simulink subsystem "T_junction"  (R2022b)
settings: Solver=VariableStepAuto  StartTime=0.0  StopTime=10.0  RelTol=1e-3
values from neighbouring files (symbols this model uses):
  C0 = 1e-5    (= 1e-05)    [plantConstants.m]
  dt = 1/samplingRate    (= 0.025)    [plantConstants.m]    (also in sysID.m)
  L0 = L_aq    [plantConstants.m]
  ni = 3    [plantConstants.m]    (also in rls_.m = no; stateEstimator.m = size(Bp,2); toPhi_.m = no; wtMod_.m = no)
  no = 3    [plantConstants.m]    (also in rls_.m = size(phi,2); stateEstimator.m = size(Cp,1); sysID.m = length(outputs); theta2ss_.m = size(y0, 1))
  Rl0 = 0    [plantConstants.m]
  Rr0 = R_aq    [plantConstants.m]
  y_max = 500*ones(2*no, 1)    [plantConstants.m]
libraries: fl_lib x6, nesl_utility x4, simulink x1
settings Model: Creator=khqc  LastModifiedBy=khqc

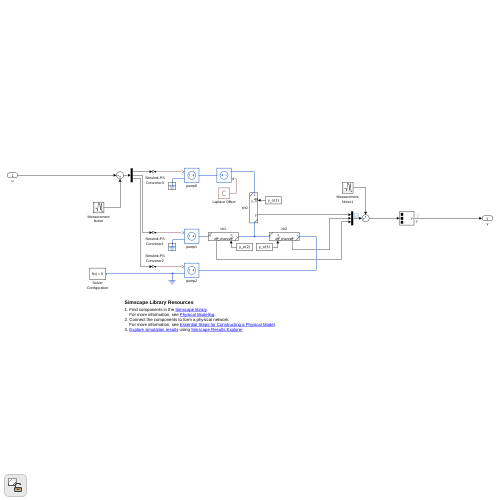
[thumbnail: Simulink's stored preview of the top-level diagram]
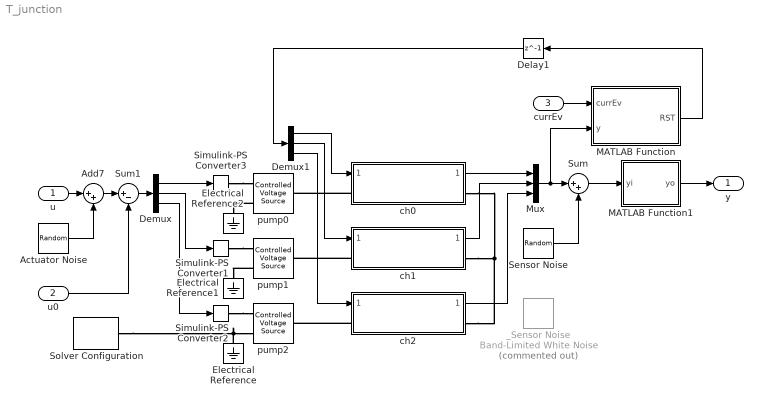
== system T_junction ==
  u : Inport
  u0 : Inport  Port=2
  currEv : Inport  Port=3
  Actuator Noise : RandomNumber  Mean=zeros(ni, 1)  Variance=0.1*ones(ni, 1)  Seed=[444; 555; 666]  SampleTime=dt  VectorParams1D=off
  Add7 : Sum  Inputs=|++
  Delay1 : Delay  DelayLength=1  InitialCondition=logical(zeros(2*no, 1))
  Demux : Demux  Outputs=3
  Demux1 : Demux  Outputs=3
  Electrical Reference : fl_lib/Electrical/Electrical Elements/Electrical Reference
  Electrical Reference1 : fl_lib/Electrical/Electrical Elements/Electrical Reference
  Electrical Reference2 : fl_lib/Electrical/Electrical Elements/Electrical Reference
  MATLAB Function : MATLAB Function  TreatAsAtomicUnit=on
  MATLAB Function1 : MATLAB Function  TreatAsAtomicUnit=on
  Mux : Mux  Inputs=3
  Sensor Noise : RandomNumber  Mean=zeros(2*no, 1)  Variance=ones(2*no, 1)  Seed=[111; 111; 222; 222; 333; 333]  SampleTime=dt  VectorParams1D=off
  Simulink-PS Converter1 : nesl_utility/Simulink-PS Converter  PhysicalDomain=network_engine_domain  SubClassName=ps_input  LeftPortType=input  RightPortType=output  PseudoPeriodic=off  Frequencies=[]  NoiseDistribution=none  NoiseParameters=[]  Unit=1  AffineConversion=off  FilteringAndDerivatives=provide  SimscapeFilterOrder=1  InputFilterTimeConstant=0.001  UdotUserProvided=0
  Simulink-PS Converter2 : nesl_utility/Simulink-PS Converter  PhysicalDomain=network_engine_domain  SubClassName=ps_input  LeftPortType=input  RightPortType=output  PseudoPeriodic=off  Frequencies=[]  NoiseDistribution=none  NoiseParameters=[]  Unit=1  AffineConversion=off  FilteringAndDerivatives=provide  SimscapeFilterOrder=1  InputFilterTimeConstant=0.001  UdotUserProvided=0
  Simulink-PS Converter3 : nesl_utility/Simulink-PS Converter  PhysicalDomain=network_engine_domain  SubClassName=ps_input  LeftPortType=input  RightPortType=output  PseudoPeriodic=off  Frequencies=[]  NoiseDistribution=none  NoiseParameters=[]  Unit=1  AffineConversion=off  FilteringAndDerivatives=provide  SimscapeFilterOrder=1  InputFilterTimeConstant=0.001  UdotUserProvided=0
  Solver Configuration : nesl_utility/Solver Configuration  PhysicalDomain=network_engine_domain  SubClassName=solver  LeftPortType=input  RightPortType=generic  Tones=[]  Harmonics=[]  SimulateNoise=off  Profile=off  UseLocalSampling=off  EnableSwitchedLinearOptims=on  FrequencyDomain=off  UseCCode=off  RelTol=0.001  AbsTol=1e-06  MinStep=1e-09  ToWorkspace=off  RevertToSquareIcSolve=off  NumHomotopyIterations=100  PhasorMode=off  PhasorModeNumHarmonics=1  ConsistencySolver=NEWTON_XTOL_AFTER_FTOL  IndexReductionMethod=DerivativeReplacement  DoDC=on  ResidualTolerance=1e-09  ConsistencyTolSource=GLOBAL  ConsistencyAbsTol=0.001  ConsistencyRelTol=0.001  ConsistencyTolFactor=0.001  UseLocalSolver=off  LocalSolverChoice=NE_BACKWARD_EULER_ADVANCER  ResolveIndetEquations=on  FunctionEvalNumThread=1  LocalSolverSampleTime=0.001  DoFixedCost=off  MaxNonlinIter=3  MaxModeIter=2  ComputeImpulses=off  ImpulseIterations=2  LinearAlgebra=auto  LinearAlgebraNumThread=0  EquationFormulation=NE_TIME_EF  DelaysMemoryBudget=1024  AutomaticFiltering=on  FilteringTimeConstant=0.001  PartitionStorageMethod=AS_NEEDED  PartitionMemoryBudget=1024  PartitionMethod=ROBUST
  Sum : Sum  Inputs=|++
  Sum1 : Sum  Inputs=|+-
  _Sensor Noise : simulink/Sources/Band-Limited White Noise  Commented=on  Cov=ones(1, 3)  Ts=dt  seed=[111 222 333]  VectorParams1D=off
  ch0 : Subsystem  ReferencedSubsystem=channel  C=C0  Rc=Rc0  L=L0*100  Rl=Rl0+0.001  R=Rr0*10  UpperSaturationLimit=2*y_max(1)  InitialCondition=0  LowerSaturationLimit=-2*y_max(1)
  ch1 : Subsystem  ReferencedSubsystem=channel  C=C0  Rc=Rc0  L=L0*100  Rl=Rl0+0.001  R=Rr0*10  UpperSaturationLimit=2*y_max(2)  InitialCondition=0  LowerSaturationLimit=-2*y_max(2)
  ch2 : Subsystem  ReferencedSubsystem=channel  C=C0  Rc=Rc0  L=L0*100  Rl=Rl0+0.001  R=Rr0*10  UpperSaturationLimit=2*y_max(3)  InitialCondition=0  LowerSaturationLimit=-2*y_max(3)
  pump0 : fl_lib/Electrical/Electrical Sources/Controlled Voltage Source
  pump1 : fl_lib/Electrical/Electrical Sources/Controlled Voltage Source
  pump2 : fl_lib/Electrical/Electrical Sources/Controlled Voltage Source
  y : Outport
  wires:
  Demux/2 -> Simulink-PS Converter1/1
  Demux/1 -> Simulink-PS Converter3/1
  Demux/3 -> Simulink-PS Converter2/1
  ch2/1 -> Mux/3
  Mux/1 -> Sum/1, MATLAB Function/2(y)
  ch1/1 -> Mux/2
  u/1 -> Add7/1
  Add7/1 -> Sum1/1
  Actuator Noise/1 -> Add7/2
  ch0/1 -> Mux/1
  u0/1 -> Sum1/2
  Sum1/1 -> Demux/1
  Sensor Noise/1 -> Sum/2
  Sum/1 -> MATLAB Function1/1(yi)
  Demux1/3 -> ch2/1
  Demux1/2 -> ch1/1
  Demux1/1 -> ch0/1
  Delay1/1 -> Demux1/1
  MATLAB Function1/1(yo) -> y/1
  MATLAB Function/1(RST) -> Delay1/1
  currEv/1 -> MATLAB Function/1(currEv)
  connections:
  Electrical Reference/LConn1 -- Solver Configuration/RConn1 -- pump2/RConn2
  ch0/RConn1 -- ch1/RConn1 -- ch2/RConn1
  Simulink-PS Converter1/RConn1 -- pump1/RConn1
  pump1/RConn2 -- Electrical Reference1/LConn1
  ch1/LConn1 -- pump1/LConn1
  pump0/RConn2 -- Electrical Reference2/LConn1
  ch2/LConn1 -- pump2/LConn1
  Simulink-PS Converter2/RConn1 -- pump2/RConn1
  Simulink-PS Converter3/RConn1 -- pump0/RConn1
  ch0/LConn1 -- pump0/LConn1

== matlab function T_junction/MATLAB Function ==
  data: currEv input Bus: event_bus; y input; RST output
function RST = simJunction(currEv, y)
% on any channel zero-crossing, reset secondary measurements to 0
persistent yp rp rstIdx;
y_ = [y(1:2:end); y(2:2:end)];
no = size(y,1);
RST = logical(zeros(no, 1));
if isempty(yp)
    yp = y_;
end
if isempty(rstIdx)
    rstIdx = 200; % 200*dt = 5 seconds
end
if isempty(rp)
    rp = currEv.r;
end

if any(rp ~= currEv.r)
    rstIdx = 200;
end

% primary zero-crossing = reset secondary
if any(currEv.r(1:no/2)) && any(sign(y_(1:no/2)) ~= sign(yp(1:no/2)))
    RST(2:2:end) = true;
else
    RST(2:2:end) = false;
end
% secondary zero-crossing = reset primary
if any(currEv.r(no/2+1:no)) && any(sign(y_(no/2+1:no)) ~= sign(yp(no/2+1:no)))
    RST(1:2:end) = true;
else
    RST(1:2:end) = false;
end
yp = y_;
rp = currEv.r;

if (rstIdx > 0)
    RST = logical(zeros(no, 1));
    rstIdx = rstIdx - 1;
end
if any(RST)
    rstIdx = 200;
end

== matlab function T_junction/MATLAB Function1 ==
  data: yi input; yo output
function yo = reshapeY(yi)
yo = [yi(1:2:end); yi(2:2:end)];
